simulink library "battery_lib"  (R2018b)
settings: Solver=VariableStepAuto  StartTime=0.0  StopTime=10.0  RelTol=1e-3
undefined symbols (not defined in the file or in its folder): DiscIntNeverNeededParam, simParams
settings Model: Creator=Taylor  LastModifiedBy=Taylor

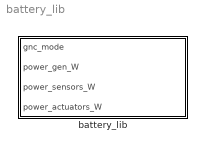
== system battery_lib ==
  battery_lib : Subsystem

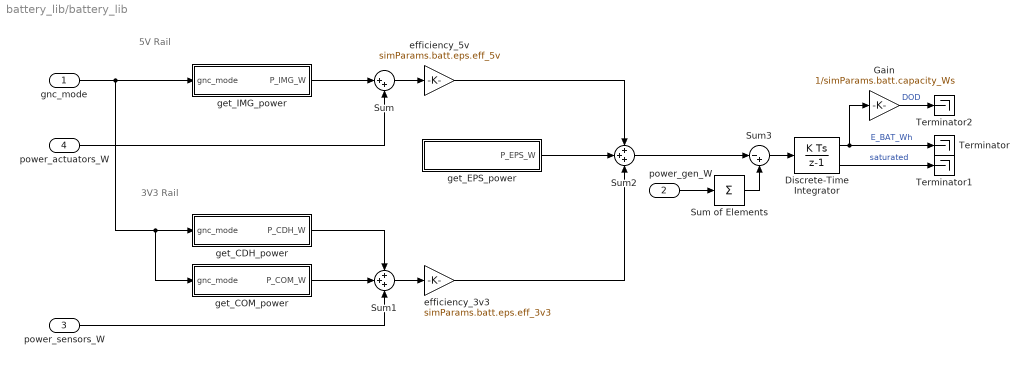
== system battery_lib/battery_lib ==
  note: 3V3 Rail
  note: 5V Rail
  gnc_mode : Inport
  power_gen_W : Inport  Port=2
  power_sensors_W : Inport  Port=3
  power_actuators_W : Inport  Port=4
  Discrete-Time Integrator : DiscreteIntegrator  InitialCondition=simParams.batt.ic.capacity_Ws  SampleTime=-1  LimitOutput=on  UpperSaturationLimit=simParams.batt.ic.capacity_Ws  LowerSaturationLimit=0  ShowSaturationPort=on  ICPrevOutput=DiscIntNeverNeededParam  ICPrevScaledInput=DiscIntNeverNeededParam
  Gain : Gain  Gain=1/simParams.batt.capacity_Ws
  Sum : Sum  Inputs=|++
  Sum of Elements : Sum  Inputs=+
  Sum1 : Sum  Inputs=+++
  Sum2 : Sum  Inputs=+++
  Sum3 : Sum  Inputs=|-+
  Terminator : Terminator
  Terminator1 : Terminator
  Terminator2 : Terminator
  "efficiency_3v3 " : Gain  Gain=simParams.batt.eps.eff_3v3
  efficiency_5v : Gain  Gain=simParams.batt.eps.eff_5v
  get_CDH_power : Subsystem
  get_COM_power : Subsystem
  get_EPS_power : Subsystem
  get_IMG_power : Subsystem
  wires:
  Sum/1 -> efficiency_5v/1
  power_actuators_W/1 -> Sum/2
  get_IMG_power/1(P_IMG_W) -> Sum/1
  "efficiency_3v3 "/1 -> Sum2/3
  Sum1/1 -> "efficiency_3v3 "/1
  get_CDH_power/1(P_CDH_W) -> Sum1/1
  power_sensors_W/1 -> Sum1/3
  get_COM_power/1(P_COM_W) -> Sum1/2
  gnc_mode/1 -> get_IMG_power/1(gnc_mode), get_COM_power/1(gnc_mode), get_CDH_power/1(gnc_mode)
  get_EPS_power/1(P_EPS_W) -> Sum2/2
  efficiency_5v/1 -> Sum2/1
  Sum2/1 -> Sum3/1
  power_gen_W/1 -> Sum of Elements/1
  Sum3/1 -> Discrete-Time Integrator/1
  Discrete-Time Integrator/1 -> Terminator/1, Gain/1  "E_BAT_Wh"
  Discrete-Time Integrator/2 -> Terminator1/1  "saturated"
  Gain/1 -> Terminator2/1  "DOD"
  Sum of Elements/1 -> Sum3/2

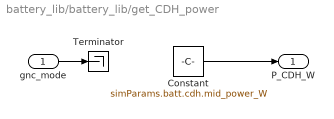
== system battery_lib/battery_lib/get_CDH_power ==
  gnc_mode : Inport
  Constant : Constant  Value=simParams.batt.cdh.mid_power_W
  Terminator : Terminator
  P_CDH_W : Outport
  wires:
  gnc_mode/1 -> Terminator/1
  Constant/1 -> P_CDH_W/1

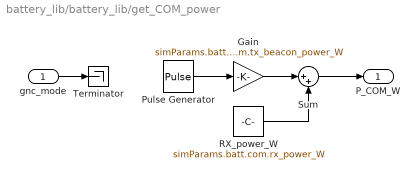
== system battery_lib/battery_lib/get_COM_power ==
  gnc_mode : Inport
  Gain : Gain  Gain=simParams.batt.com.tx_beacon_power_W
  Pulse Generator : DiscretePulseGenerator  PulseType=Time based  Period=60  PulseWidth=5
  RX_power_W : Constant  Value=simParams.batt.com.rx_power_W
  Sum : Sum  Inputs=|++
  Terminator : Terminator
  P_COM_W : Outport
  wires:
  gnc_mode/1 -> Terminator/1
  Pulse Generator/1 -> Gain/1
  Gain/1 -> Sum/1
  RX_power_W/1 -> Sum/2
  Sum/1 -> P_COM_W/1

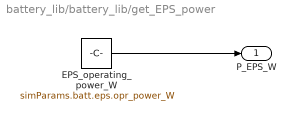
== system battery_lib/battery_lib/get_EPS_power ==
  EPS_operating_power_W : Constant  Value=simParams.batt.eps.opr_power_W
  P_EPS_W : Outport
  wires:
  EPS_operating_power_W/1 -> P_EPS_W/1

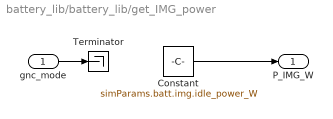
== system battery_lib/battery_lib/get_IMG_power ==
  gnc_mode : Inport
  Constant : Constant  Value=simParams.batt.img.idle_power_W
  Terminator : Terminator
  P_IMG_W : Outport
  wires:
  gnc_mode/1 -> Terminator/1
  Constant/1 -> P_IMG_W/1
